simulink model "A1"  (R2021a)
settings: Solver=VariableStepAuto  StartTime=0.0  StopTime=10.0  RelTol=1e-3
settings Model: Creator=KAVITA KUMARI  LastModifiedBy=KAVITA KUMARI

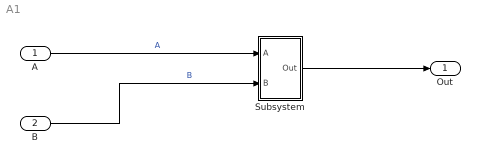
== system A1 ==
  A : Inport
  B : Inport  Port=2
  Subsystem : Subsystem
  Out : Outport
  wires:
  A/1 -> Subsystem/1(A)  "A"
  B/1 -> Subsystem/2(B)  "B"
  Subsystem/1(Out) -> Out/1

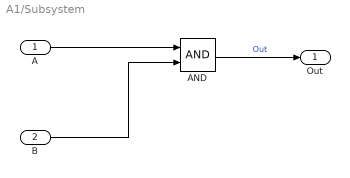
== system A1/Subsystem ==
  A : Inport
  B : Inport  Port=2
  AND : Logic  AllPortsSameDT=off  OutDataTypeStr=boolean
  Out : Outport
  wires:
  B/1 -> AND/2
  AND/1 -> Out/1  "Out"
  A/1 -> AND/1
